simulink model "p5p5e_model"  (Simulink 8.9)
settings: Solver=ode45  StartTime=0.0  StopTime=2000  RelTol=1e-3  EnableMultiTasking=on
undefined symbols (not defined in the file or in its folder): Kpd, T_d, T_f
undefined symbols (not defined in the file): data
libraries: simulink x2
settings Model: Creator=markh  LastModifiedBy=marmad
settings DataIOCC: SignalLoggingName=sigsOut
settings OptimizationCC: InitFltsAndDblsToZero=on
settings DebuggingCC: SaveWithParameterizedLinksMsg=none  SignalResolutionControl=TryResolveAllWithWarning  MultiTaskDSMMsg=warning  MultiTaskCondExecSysMsg=none
settings HardwareCC: TargetUnknown=on
settings GRTTargetCC: TargetFcnLib=ansi_tfl_tmw.mat

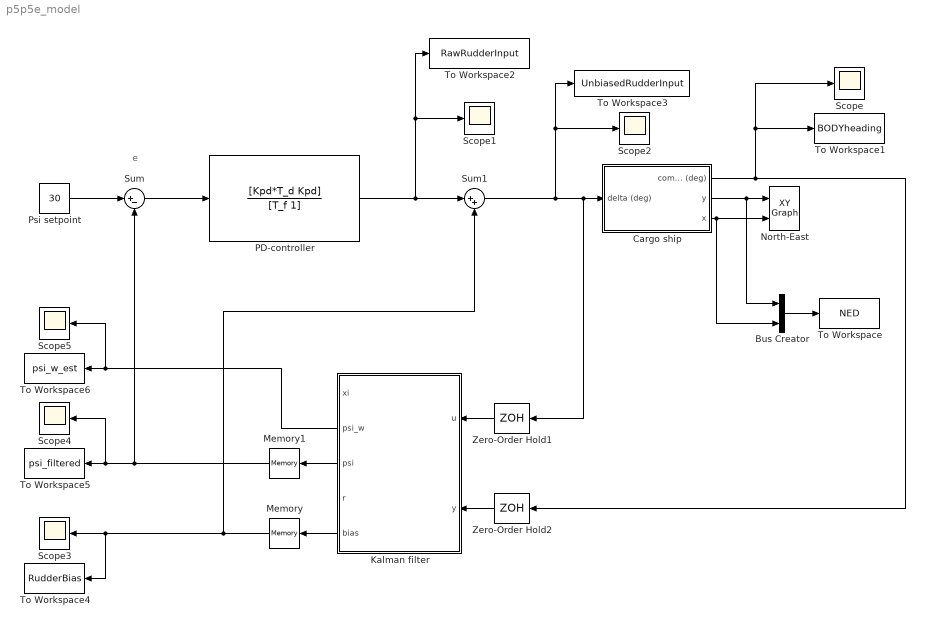
== system p5p5e_model ==
  note: e
  Bus Creator : BusCreator  Inputs=2
  Cargo ship : Subsystem  mask(Simple shipmodel for a cargo ship){noise=on, current=on, logic=on}
      mask prompts: noise "measurement noise"; logic "waves"
      mask help:
      | Measurement noise:
      | 	checked = noise on
      | 	unchecked = noise off
      |
      | Current:
      | 	checked = current on
      | 	unchecked = current off
      |
      | Waves:
      | 	checked = waves on
      | 	unchecked = waves off
      |
      | Author: Jørgen Spjøtvold, 9/10-2003
      | TTK 4115 Linear system theory.
      | Modified by Jostein Bakkeheim 26/10-2006
  Kalman filter : MATLAB Function  TreatAsAtomicUnit=on  mask{data=data}
      mask prompts: data "data struct"
  Memory : Memory  InheritSampleTime=on
  Memory1 : Memory  InheritSampleTime=on
  North-East : simulink/Sinks/XY Graph  xmin=-5000  xmax=7000  ymin=-5000  ymax=5000  st=-1
  PD-controller : TransferFcn  Numerator=[Kpd*T_d Kpd]  Denominator=[T_f 1]
  Psi setpoint : Constant  Value=30
  Scope{,1..5} (6 alike) : Scope
  Sum : Sum  Inputs=|+-
  Sum1 : Sum  Inputs=|++
  To Workspace : ToWorkspace  VariableName=NED  SaveFormat=Timeseries  SampleTime=-1
  To Workspace1 : ToWorkspace  VariableName=BODYheading  SaveFormat=Timeseries  SampleTime=-1
  To Workspace2 : ToWorkspace  VariableName=RawRudderInput  SaveFormat=Timeseries  SampleTime=-1
  To Workspace3 : ToWorkspace  VariableName=UnbiasedRudderInput  SaveFormat=Timeseries  SampleTime=-1
  To Workspace4 : ToWorkspace  VariableName=RudderBias  SaveFormat=Timeseries  SampleTime=-1
  To Workspace5 : ToWorkspace  VariableName=psi_filtered  SaveFormat=Timeseries  SampleTime=-1
  To Workspace6 : ToWorkspace  VariableName=psi_w_est  SaveFormat=Timeseries  SampleTime=-1
  Zero-Order Hold1 : ZeroOrderHold  SampleTime=0.1
  Zero-Order Hold2 : ZeroOrderHold  SampleTime=0.1
  wires:
  Cargo ship/3(x) -> North-East/2, Bus Creator/2
  Cargo ship/2(y) -> Bus Creator/1, North-East/1
  Cargo ship/1(compass (deg)) -> To Workspace1/1, Scope/1, Zero-Order Hold2/1
  Bus Creator/1 -> To Workspace/1
  Psi setpoint/1 -> Sum/1
  Sum/1 -> PD-controller/1
  Zero-Order Hold1/1 -> Kalman filter/1(u)
  Zero-Order Hold2/1 -> Kalman filter/2(y)
  PD-controller/1 -> Sum1/1, To Workspace2/1, Scope1/1
  Kalman filter/5(bias) -> Memory/1
  Kalman filter/3(psi) -> Memory1/1
  Memory/1 -> Sum1/2, To Workspace4/1, Scope3/1
  Memory1/1 -> Sum/2, Scope4/1, To Workspace5/1
  Sum1/1 -> Zero-Order Hold1/1, Cargo ship/1(delta (deg)), Scope2/1, To Workspace3/1
  Kalman filter/2(psi_w) -> Scope5/1, To Workspace6/1

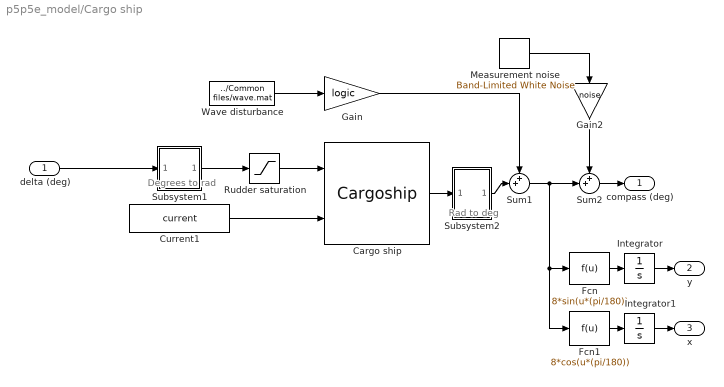
== system p5p5e_model/Cargo ship ==
  note: Degrees to rad
  note: Rad to deg
  delta (deg) : Inport
  Cargo ship : S-Function  FunctionName=Cargoship  SFunctionDeploymentMode=off  EnableBusSupport=off  mask(Cargo ship){}
      mask help:
      | S-function which simulates a cargo ship.
      |
      | Author: Jørgen Spjøtvold
      | 20.10-2003
      | Modified by Jostein Bakkeheim 27.10.2006
  Current1 : Constant  Value=current
  Fcn : Fcn  Expr=8*sin(u*(pi/180))
  Fcn1 : Fcn  Expr=8*cos(u*(pi/180))
  Gain : Gain  Gain=logic  SaturateOnIntegerOverflow=on  OutDataTypeStr=Inherit: Same as input  ParamDataTypeStr=Inherit: Same as input
  Gain2 : Gain  Gain=noise  SaturateOnIntegerOverflow=on  OutDataTypeStr=Inherit: Same as input  ParamDataTypeStr=Inherit: Same as input
  Integrator : Integrator
  Integrator1 : Integrator
  Measurement noise : simulink/Sources/Band-Limited White Noise  Cov=[0.001]  Ts=.5  seed=[23341]
  Rudder saturation : Saturate  UpperLimit=45*(pi/180)  LowerLimit=-45*(pi/180)
  Subsystem1 : Subsystem  mask(degrees to radians){}
      mask help: Converts degrees to radians
      mask Display: fprintf('D2R');
  Subsystem2 : Subsystem  mask(radians to degrees){}
      mask help: Converts radians to degrees
      mask Display: fprintf('R2D');
  Sum1 : Sum  Inputs=++|  SaturateOnIntegerOverflow=on
  Sum2 : Sum  Inputs=++|  SaturateOnIntegerOverflow=on
  Wave disturbance : FromFile  FileName=../Common files/wave.mat  SampleTime=0
  compass (deg) : Outport
  y : Outport  Port=2
  x : Outport  Port=3
  wires:
  delta (deg)/1 -> Subsystem1/1(In1)
  Fcn/1 -> Integrator/1
  Integrator/1 -> y/1
  Fcn1/1 -> Integrator1/1
  Integrator1/1 -> x/1
  Wave disturbance/1 -> Gain/1
  Subsystem2/1(Out1) -> Sum1/2
  Gain/1 -> Sum1/1
  Sum1/1 -> Fcn/1, Fcn1/1, Sum2/2
  Cargo ship/1 -> Subsystem2/1(In1)
  Subsystem1/1(Out1) -> Rudder saturation/1
  Rudder saturation/1 -> Cargo ship/1
  Sum2/1 -> compass (deg)/1
  Measurement noise/1 -> Gain2/1
  Gain2/1 -> Sum2/1
  Current1/1 -> Cargo ship/2

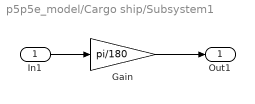
== system p5p5e_model/Cargo ship/Subsystem1 ==
  In1 : Inport
  Gain : Gain  Gain=pi/180  SaturateOnIntegerOverflow=on  OutDataTypeStr=Inherit: Same as input  ParamDataTypeStr=Inherit: Same as input
  Out1 : Outport
  wires:
  Gain/1 -> Out1/1
  In1/1 -> Gain/1

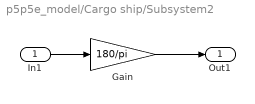
== system p5p5e_model/Cargo ship/Subsystem2 ==
  In1 : Inport
  Gain : Gain  Gain=180/pi  SaturateOnIntegerOverflow=on  OutDataTypeStr=Inherit: Same as input  ParamDataTypeStr=Inherit: Same as input
  Out1 : Outport
  wires:
  Gain/1 -> Out1/1
  In1/1 -> Gain/1

== matlab function Kalman filter ==
  settings: updateMethod=DISCRETE  sampleTime=Ts
  data: xi output double; psi_w output double; u input double; psi output double; r output double; y input double; data parameter double; bias output double
function [xi, psi_w, psi, r, bias] = fcn(u,y,data)
persistent xpri xhat P;

A = data.A;
B = data.B;
C = data.C;
Q = data.Q;
R = data.R;
I = data.I;
if isempty(xpri)
    xpri = data.xhat0;
    P = data.P;
end

K = P*C'/(C*P*C' + R);
xhat = xpri + K*(y - C*xpri);
P = (I - K*C)*P*(I - K*C)' + K*R*K';

xpri = A*xhat + B*u;
P = A*P*A' + Q;

xi = xhat(1);
psi_w = xhat(2);
psi = xhat(3);
r = xhat(4);
bias = xhat(5);
